simulink model "counter"  (R2020b)
settings: Solver=VariableStepAuto  StartTime=0.0  StopTime=10.0  RelTol=1e-3
settings Model: Creator=JAGRUTI SHINDE  LastModifiedBy=JAGRUTI SHINDE

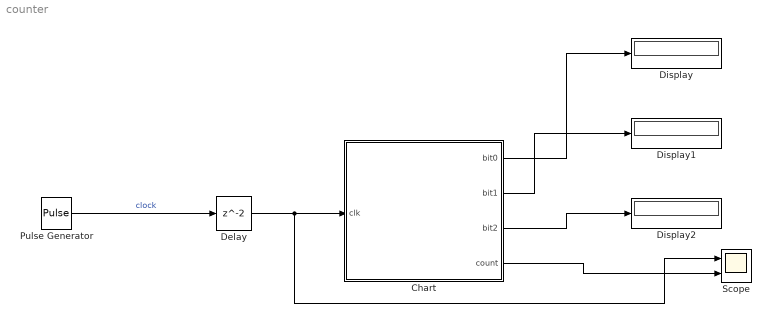
== system counter ==
  Chart : Stateflow chart  TreatAsAtomicUnit=on
  Delay : Delay
  Display : Display
  Display1 : Display
  Display2 : Display
  Pulse Generator : DiscretePulseGenerator  PulseType=Time based  PulseWidth=50
  Scope : Scope  NumInputPorts=2
  wires:
  Pulse Generator/1 -> Delay/1  "clock"
  Chart/1(bit0) -> Display/1
  Chart/2(bit1) -> Display1/1
  Chart/3(bit2) -> Display2/1
  Chart/4(count) -> Scope/2
  Delay/1 -> Scope/1, Chart/1(clk)

== stateflow chart counter/Chart ==
  state State_0
    entry:
    bit0=0;
    bit1=0;
    bit2=0;
    exit:
    count=0;
  state State_1
    entry:
    bit0=1;
    bit1=0;
    bit2=0;
    exit:
    count=1;
  state State_4
    entry:
    bit0=0;
    bit1=0;
    bit2=1;
    exit:
    count=4;
  state State_2
    entry:
    bit0=0;
    bit1=1;
    bit2=0;
    exit:
    count=2;
  state State_3
    entry:
    bit0=1;
    bit1=1;
    bit2=0;
    exit:
    count=3;
  (default) -> State_0
  State_0 -> State_1 : [clk==1]
  State_4 -> State_0 : [clk==1]
  State_1 -> State_2 : [clk==1]
  State_3 -> State_4 : [clk==1]
  State_2 -> State_3 : [clk==1]
  data: bit0 output; bit1 output; bit2 output; count output; clk input
